simulink model "frst"  (Simulink 7.4)
settings: Solver=ode45  StartTime=0.0  StopTime=10.0  RelTol=1e-3
settings Model: Creator=autologin  LastModifiedBy=autologin

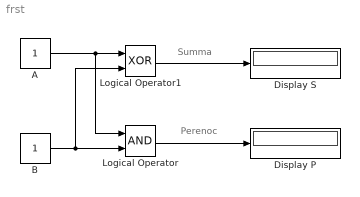
== system frst ==
  note: Summa
  note: Perenoc
  A : Constant  OutDataType=fixdt(1, 16)  OutScaling=2^0
  B : Constant  OutDataType=fixdt(1, 16)  OutScaling=2^0
  Display P : Display
  Display S : Display
  Logical Operator : Logic  AllPortsSameDT=off  OutDataTypeMode=boolean  LogicDataType=fixdt(0, 8)  OutDataTypeStr=boolean
  Logical Operator1 : Logic  Operator=XOR  AllPortsSameDT=off  OutDataTypeMode=boolean  LogicDataType=fixdt(0, 8)  OutDataTypeStr=boolean
  wires:
  A/1 -> Logical Operator1/1, Logical Operator/1
  B/1 -> Logical Operator/2, Logical Operator1/2
  Logical Operator1/1 -> Display S/1
  Logical Operator/1 -> Display P/1
